simulink model "ProjectArchitecture"  (R2026a)
settings: Solver=VariableStepAuto  StopTime=100
undefined symbols (not defined in the file): Boomgate_Up, Close_Cmd, Dwn, Open, Pedestrian_Lights_On, Traffic_Lights_On
(part 2 of 2)

== system ProjectArchitecture/TrafficManagmentSystem/Control(Optional)/R//W_Status ==
  Bus Element In1 : Inport  PortName=Node_Status_Msg
  Bus Element Out1 : Outport  PortName=Node_Status_GUI
  Bus Element Out2 : Outport  Port=2  PortName=Node_Not_Responding

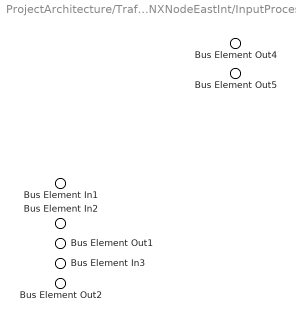
== system ProjectArchitecture/TrafficManagmentSystem/QNXNodeEastInt/InputProcessing ==
  Bus Element In1 : Inport  PortName=ENode_NetBusIn
  Bus Element In2 : Inport  Port=2  PortName=Node_PedBtnEastBus
  Bus Element In3 : Inport  Port=3  PortName=Node_VehSensEastBus
  Bus Element Out4 : Outport  PortName=Force_Phase_Command
  Bus Element Out5 : Outport  Port=2  PortName=Failure_Detected
  Bus Element Out1 : Outport  Port=3  PortName=Pedestrian_Button
  Bus Element Out2 : Outport  Port=4  PortName=Vehicle_Precence

== system ProjectArchitecture/TrafficManagmentSystem/QNXNodeEastInt/OutputProcessing ==
  Bus Element In1 : Inport  PortName=Train_Node_Status
  Bus Element In2 : Inport  Port=2  PortName=Pedestrian_Lights_On/Off
  Bus Element In3 : Inport  Port=3  PortName=Traffic_Lights_On/Off
  Bus Element Out1 : Outport  PortName=Node_PedLtEastBus
  Bus Element Out2 : Outport  Port=2  PortName=Node_TrLtEastBus
  Bus Element Out3 : Outport  Port=3  PortName=ENode_NetBusOut

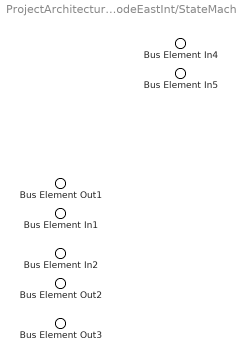
== system ProjectArchitecture/TrafficManagmentSystem/QNXNodeEastInt/StateMachine ==
  Bus Element In4 : Inport  PortName=Force_Phase_Command
  Bus Element In5 : Inport  Port=2  PortName=Failure_Detected
  Bus Element In1 : Inport  Port=3  PortName=Pedestrian_Button
  Bus Element In2 : Inport  Port=4  PortName=Vehicle_Precence
  Bus Element Out1 : Outport  PortName=Current_State
  Bus Element Out2 : Outport  Port=2  PortName=Pedestrian_Lights_On/Off
  Bus Element Out3 : Outport  Port=3  PortName=Traffic_Lights_On/Off

== system ProjectArchitecture/TrafficManagmentSystem/QNXNodeEastInt/StatusUpdate ==
  Bus Element In1 : Inport  PortName=Current_State
  Bus Element Out1 : Outport  PortName=Train_Node_Status

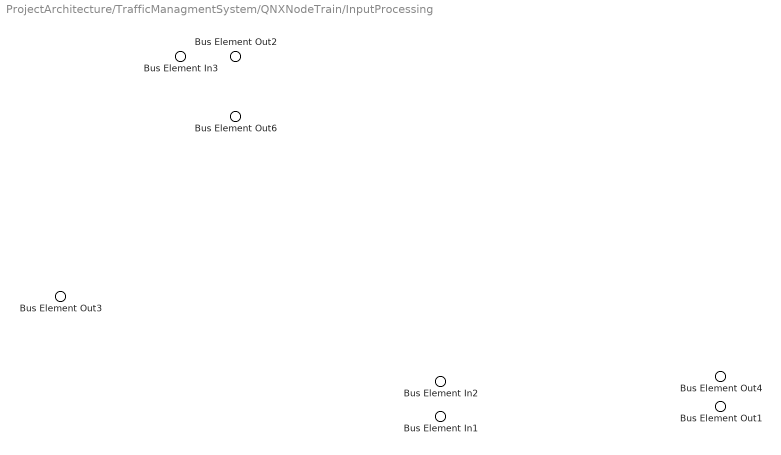
== system ProjectArchitecture/TrafficManagmentSystem/QNXNodeTrain/InputProcessing ==
  Bus Element In3 : Inport  PortName=Node_TrainBmGtPos
  Bus Element In1 : Inport  Port=2  PortName=Node_TrainSensBus
  Bus Element In2 : Inport  Port=3  PortName=TNode_NetBusIn
  Bus Element Out2 : Outport  PortName=Force_Phase_Command
  Bus Element Out6 : Outport  Port=2  PortName=Failure_Detected
  Bus Element Out4 : Outport  Port=3  PortName=Train_passed_Sensor
  Bus Element Out1 : Outport  Port=4  PortName=Train_Approach_Sensor
  Bus Element Out3 : Outport  Port=5  PortName=Boomgate_Position

== system ProjectArchitecture/TrafficManagmentSystem/QNXNodeTrain/OutputProcessing ==
  Bus Element In4 : Inport  PortName=Train_Node_Heartbeat
  Bus Element In2 : Inport  Port=2  PortName=Boomgate_Up/Dwn
  Bus Element In3 : Inport  Port=3  PortName=Warning_signals
  Bus Element In1 : Inport  Port=4  PortName=Warning_Sound
  Bus Element Out2 : Outport  PortName=Node_TrainSigBmGt
  Bus Element Out1 : Outport  Port=2  PortName=Node_TrainSigBus
  Bus Element Out3 : Outport  Port=3  PortName=TNode_NetBusOut

== system ProjectArchitecture/TrafficManagmentSystem/QNXNodeTrain/State machine timing manager (extra) ==

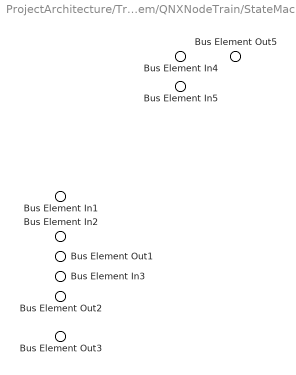
== system ProjectArchitecture/TrafficManagmentSystem/QNXNodeTrain/StateMachine ==
  Bus Element In5 : Inport  PortName=Force_Phase_Command
  Bus Element In4 : Inport  Port=2  PortName=Failure_Detected
  Bus Element In1 : Inport  Port=3  PortName=Train_passed_Sensor
  Bus Element In2 : Inport  Port=4  PortName=Train_Approach_Sensor
  Bus Element In3 : Inport  Port=5  PortName=Boomgate_Position
  Bus Element Out5 : Outport  PortName=Current_State
  Bus Element Out1 : Outport  Port=2  PortName=Boomgate_Up/Dwn
  Bus Element Out2 : Outport  Port=3  PortName=Warning_signals
  Bus Element Out3 : Outport  Port=4  PortName=Warning_Sound

== system ProjectArchitecture/TrafficManagmentSystem/QNXNodeTrain/StatusUpdate ==
  Bus Element In1 : Inport  PortName=Current_State
  Bus Element Out1 : Outport  PortName=Train_Node_Status

== system ProjectArchitecture/TrafficManagmentSystem/QNXNodeWestInt/InputProcessing ==
  Bus Element In1 : Inport  PortName=Node_PedBtnWestBus
  Bus Element In2 : Inport  Port=2  PortName=Node_VehSensWestBus
  Bus Element In3 : Inport  Port=3  PortName=WNode_NetBusIn
  Bus Element Out4 : Outport  PortName=Force_Phase_Command
  Bus Element Out5 : Outport  Port=2  PortName=Failure_Detected
  Bus Element Out1 : Outport  Port=3  PortName=Pedestrian_Button
  Bus Element Out2 : Outport  Port=4  PortName=Vehicle_Precence

== system ProjectArchitecture/TrafficManagmentSystem/QNXNodeWestInt/OutputProcessing ==
  Bus Element In1 : Inport  PortName=Train_Node_Status
  Bus Element In2 : Inport  Port=2  PortName=Pedestrian_Lights_On/Off
  Bus Element In3 : Inport  Port=3  PortName=Traffic_Lights_On/Off
  Bus Element Out1 : Outport  PortName=Node_PedLtWestBus
  Bus Element Out2 : Outport  Port=2  PortName=Node_TrLtWestBus
  Bus Element Out3 : Outport  Port=3  PortName=WNode_NetBusOut

== system ProjectArchitecture/TrafficManagmentSystem/QNXNodeWestInt/StateMachine ==
  Bus Element In4 : Inport  PortName=Force_Phase_Command
  Bus Element In5 : Inport  Port=2  PortName=Failure_Detected
  Bus Element In1 : Inport  Port=3  PortName=Pedestrian_Button
  Bus Element In2 : Inport  Port=4  PortName=Vehicle_Precence
  Bus Element Out1 : Outport  PortName=Current_State
  Bus Element Out2 : Outport  Port=2  PortName=Pedestrian_Lights_On/Off
  Bus Element Out3 : Outport  Port=3  PortName=Traffic_Lights_On/Off

== system ProjectArchitecture/TrafficManagmentSystem/QNXNodeWestInt/StatusUpdate ==
  Bus Element In1 : Inport  PortName=Current_State
  Bus Element Out1 : Outport  PortName=Train_Node_Status

== system ProjectArchitecture/TrafficManagmentSystem/UserInterface/InputProcessing ==
  Bus Element In1 : Inport  PortName=CNode_NetBusIn
  Bus Element Out1 : Outport  PortName=Display_Info

== system ProjectArchitecture/TrafficManagmentSystem/UserInterface/Interface (TBD) ==
  Bus Element In1 : Inport  PortName=Display_Info
  Bus Element Out1 : Outport  PortName=Current_State
  Bus Element Out2 : Outport  Port=2  PortName=Command_Out

== system ProjectArchitecture/TrafficManagmentSystem/UserInterface/OutputProcessing ==
  Bus Element In1 : Inport  PortName=UsrInt_Node_Status
  Bus Element In2 : Inport  Port=2  PortName=Command_Out
  Bus Element Out1 : Outport  PortName=CNode_NetBusOut

== system ProjectArchitecture/TrafficManagmentSystem/UserInterface/StatusUpdate ==
  Bus Element In1 : Inport  PortName=Current_State
  Bus Element Out1 : Outport  PortName=UsrInt_Node_Status
